simulink model "MRACSBR"  (R2022b)
settings: Solver=FixedStepAuto  StartTime=0.0  StopTime=inf  FixedStep=0.01  RelTol=1e-3
undefined symbols (not defined in the file): b
libraries: arduinolib x4, arduinosensorlib x1
settings Model: SimulationMode=external  ExtModeTrigDuration=2  Creator=edgar  LastModifiedBy=Sayan
settings SolverCC: AllowMultiTaskInputOutput=on  AutoInsertRateTranBlk=on
settings OptimizationCC: EnhancedBackFolding=on  PassReuseOutputArgsAs=Individual arguments  ZeroExternalMemoryAtStartup=off  ZeroInternalMemoryAtStartup=off  MaxStackSize=64  OptimizeBlockOrder=speed  DifferentSizesBufferReuse=on  OptimizationCustomize=off  EfficientTunableParamExpr=on
settings DebuggingCC: ParameterTunabilityLossMsg=error
settings HardwareCC: ProdBitPerInt=16  ProdBitPerPointer=16  ProdBitPerSizeT=16  ProdBitPerPtrDiffT=16  ProdLargestAtomicFloat=None  ProdWordSize=8  ProdLongLongMode=on  ProdHWDeviceType=Atmel->AVR  UseEmbeddedCoderFeatures=off  UseSimulinkCoderFeatures=off
settings ModelReferenceCC: EnableRefExpFcnMdlSchedulingChecks=on
settings SFSimCC: MATLABDynamicMemAlloc=off
settings RTWCC: Description=Embedded Coder  SystemTargetFile=ert.tlc  HardwareBoard=Arduino Uno  TemplateMakefile=ert_default_tmf  RTWVerbose=off  Toolchain=Arduino AVR  BuildConfiguration=Faster Runs
settings CodeAppCC: ForceParamTrailComments=on  OperatorAnnotations=on  SimulinkDataObjDesc=on  SFDataObjDesc=on  MangleLength=10  InsertBlockDesc=on
settings ERTTargetCC: SupportContinuousTime=on  SupportNonInlinedSFcns=on  SupportVariableSizeSignals=on  ExtMode=on  ExtModeTransport=3  ExtModeStaticAlloc=on  ExtModeAutomaticAllocSize=off  ExtModeStaticAllocSize=250  ExtModeMexFile=ext_xcp  ExtModeMexArgs=0 3 115200  ExtModeIntrfLevel=Level2 - Open  ERTSrcFileBannerTemplate=codertarget_code_template.cgt  ERTHdrFileBannerTemplate=codertarget_code_template.cgt  ERTDataSrcFileTemplate=codertarget_code_template.cgt  ERTDataHdrFileTemplate=codertarget_code_template.cgt

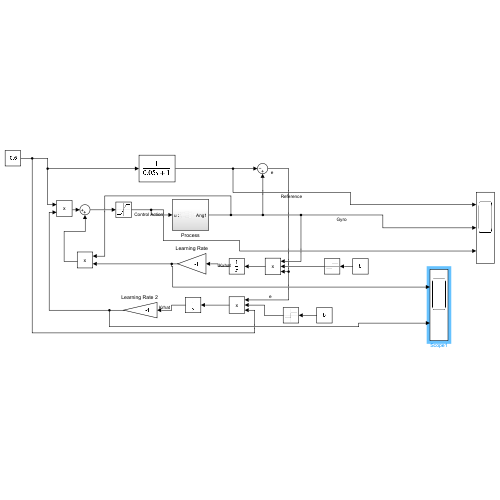
[thumbnail: Simulink's stored preview of the top-level diagram]
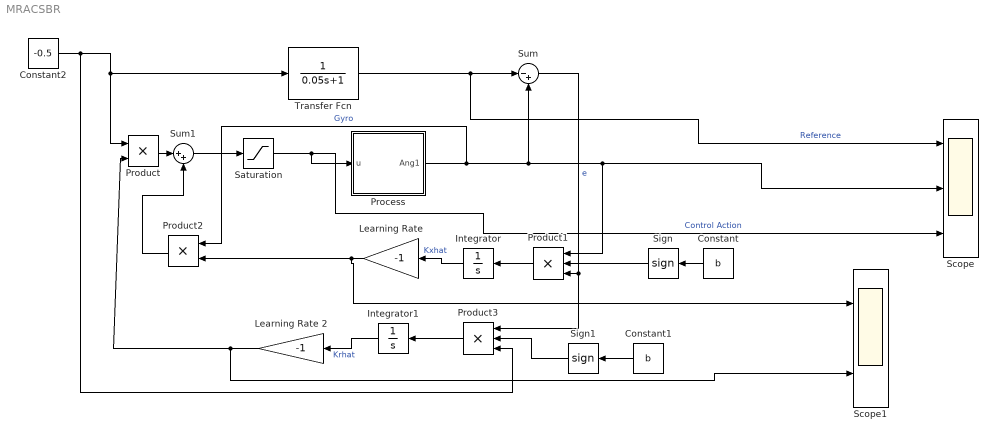
== system MRACSBR ==
  Constant : Constant  Value=b
  Constant1 : Constant  Value=b
  Constant2 : Constant  Value=-0.5
  Integrator : Integrator  InitialCondition=-15  UpperSaturationLimit=1000  LowerSaturationLimit=-1000
  Integrator1 : Integrator  InitialCondition=15  UpperSaturationLimit=1000  LowerSaturationLimit=-1000  AbsoluteTolerance=-1
  Learning Rate : Gain  Gain=-1
  "Learning Rate 2 " : Gain  Gain=-1
  Process : Subsystem
  Product : Product
  Product1 : Product  Inputs=3
  Product2 : Product
  Product3 : Product  Inputs=3
  Saturation : Saturate  UpperLimit=255  LowerLimit=-255
  Scope : Scope  NumInputPorts=3
  Scope1 : Scope  NumInputPorts=2
  Sign : Signum
  Sign1 : Signum
  Sum : Sum  Inputs=|-+
  Sum1 : Sum  Inputs=|++
  Transfer Fcn : TransferFcn  Denominator=[0.05 1]
  wires:
  Sum1/1 -> Saturation/1
  Product/1 -> Sum1/1
  Constant/1 -> Sign/1
  Product1/1 -> Integrator/1
  Integrator/1 -> Learning Rate/1  "Kxhat"
  Constant1/1 -> Sign1/1
  Integrator1/1 -> "Learning Rate 2 "/1  "Krhat"
  Product3/1 -> Integrator1/1
  Product2/1 -> Sum1/2
  Sign/1 -> Product1/2
  Sum/1 -> Product3/1, Product1/3  "e"
  Sign1/1 -> Product3/2
  Saturation/1 -> Process/1(u), Scope/3  "Control Action"
  Process/1(Ang1) -> Product2/1, Sum/2, Product1/1, Scope/2  "Gyro"
  Transfer Fcn/1 -> Scope/1, Sum/1  "Reference"
  Constant2/1 -> Product3/3, Product/1, Transfer Fcn/1
  Learning Rate/1 -> Product2/2, Scope1/1
  "Learning Rate 2 "/1 -> Product/2, Scope1/2

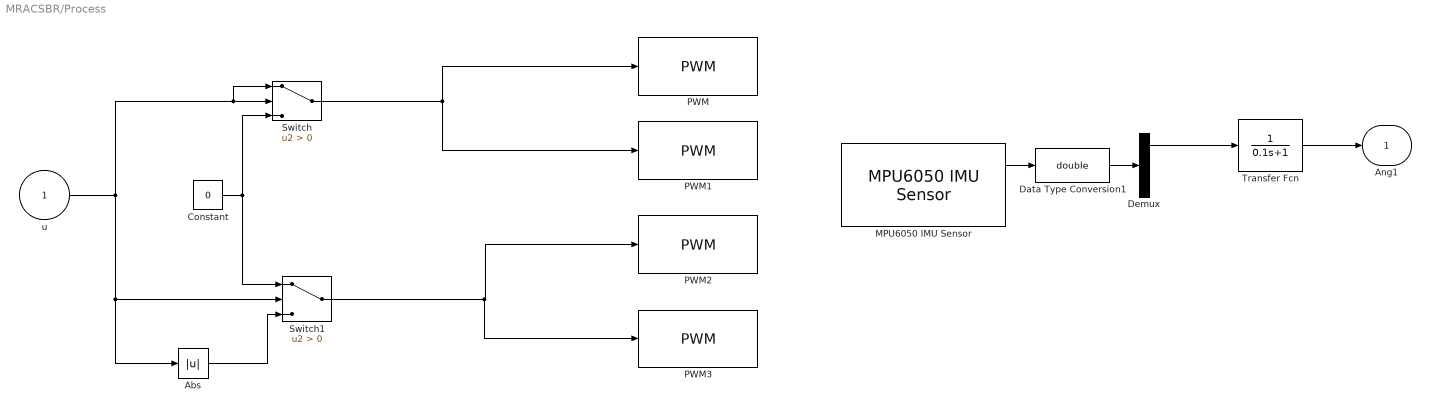
== system MRACSBR/Process ==
  u : Inport
  Abs : Abs  SaturateOnIntegerOverflow=off
  Constant : Constant  Value=0
  Data Type Conversion1 : DataTypeConversion  OutDataTypeStr=double  SaturateOnIntegerOverflow=off  RndMeth=Floor
  Demux : Demux  Outputs=3
  MPU6050 IMU Sensor : arduinosensorlib/MPU6050 IMU Sensor  SlaveAddress=0x68  Accel=on  AngularRate=on  Temperature=off  Status=off  Timestamp=off  EulerAngles=off  Quat=off  AccelRange=4G  GyroRange=500 dps  DmpOdr=200 Hz  Dlpf=Accelerometer: 260Hz, Gyroscope: 256Hz  spf=1  SampleTime=-1  QueueSizeFactor=1
  PWM : arduinolib/PWM  pinNumber=11  frequencyType=Default  desiredFrequency=490.2  achievableFrequency=490.2
  PWM1 : arduinolib/PWM  pinNumber=6  frequencyType=Default  desiredFrequency=490.2  achievableFrequency=490.2
  PWM2 : arduinolib/PWM  pinNumber=10  frequencyType=Default  desiredFrequency=490.2  achievableFrequency=490.2
  PWM3 : arduinolib/PWM  pinNumber=5  frequencyType=Default  desiredFrequency=490.2  achievableFrequency=490.2
  Switch : Switch  Criteria=u2 > Threshold  SaturateOnIntegerOverflow=off  InputSameDT=off
  Switch1 : Switch  Criteria=u2 > Threshold  SaturateOnIntegerOverflow=off  InputSameDT=off
  Transfer Fcn : TransferFcn  Denominator=[0.1 1]
  Ang1 : Outport
  wires:
  Constant/1 -> Switch/3, Switch1/1
  MPU6050 IMU Sensor/1 -> Data Type Conversion1/1
  Switch1/1 -> PWM3/1, PWM2/1
  u/1 -> Switch1/2, Abs/1, Switch/1, Switch/2
  Abs/1 -> Switch1/3
  Demux/1 -> Transfer Fcn/1
  Switch/1 -> PWM1/1, PWM/1
  Transfer Fcn/1 -> Ang1/1
  Data Type Conversion1/1 -> Demux/1
